simulink model "LFC_isolated_area"  (R2014a)
settings: Solver=ode45  StartTime=0.0  StopTime=25  RelTol=1e-3
libraries: cstblocks x4
settings Model: Creator=Divya M  LastModifiedBy=Divya M

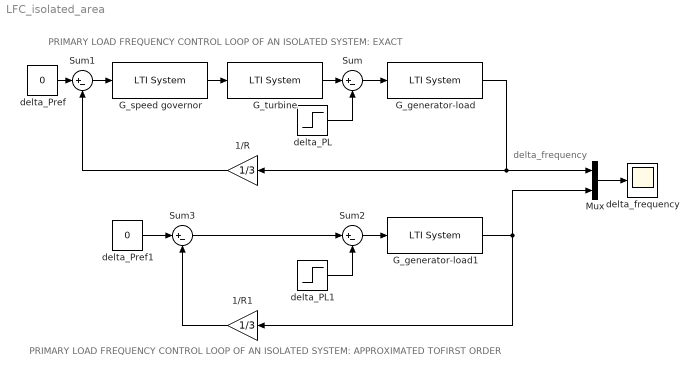
== system LFC_isolated_area ==
  note: PRIMARY LOAD FREQUENCY CONTROL LOOP OF AN ISOLATED SYSTEM: APPROXIMATED TOFIRST ORDER
  note: PRIMARY LOAD FREQUENCY CONTROL LOOP OF AN ISOLATED SYSTEM: EXACT
  note: delta_frequency
  1/R : Gain  Gain=1/3
  1/R1 : Gain  Gain=1/3
  G_generator-load : cstblocks/LTI System  sys=tf(100,[20 1])  IC=[]
  G_generator-load1 : cstblocks/LTI System  sys=tf(100,[20 1])  IC=[]
  G_speed governor : cstblocks/LTI System  sys=tf(10,[0.4 1])  IC=[]
  G_turbine : cstblocks/LTI System  sys=tf(0.1,[0.5 1])  IC=[]
  Mux : Mux  Inputs=2
  Sum{,1..3} (4 alike) : Sum  Inputs=|+-
  delta_PL : Step  After=0.01  SampleTime=0
  delta_PL1 : Step  After=0.01  SampleTime=0
  delta_Pref : Constant  Value=0
  delta_Pref1 : Constant  Value=0
  delta_frequency : Scope
      settings: YMin=-0.05  YMax=0.005
  wires:
  delta_Pref/1 -> Sum1/1
  Sum1/1 -> G_speed governor/1
  G_speed governor/1 -> G_turbine/1
  G_turbine/1 -> Sum/1
  Sum/1 -> G_generator-load/1
  G_generator-load/1 -> 1/R/1, Mux/1
  delta_PL/1 -> Sum/2
  1/R/1 -> Sum1/2
  delta_Pref1/1 -> Sum3/1
  Sum2/1 -> G_generator-load1/1
  G_generator-load1/1 -> Mux/2, 1/R1/1
  delta_PL1/1 -> Sum2/2
  1/R1/1 -> Sum3/2
  Sum3/1 -> Sum2/1
  Mux/1 -> delta_frequency/1
